simulink model "oxigeno"  (Simulink 7.5)
settings: Solver=ode45  StartTime=0.0  StopTime=10.0  RelTol=1e-3
settings Model: Creator=My Laptop  LastModifiedBy=My Laptop

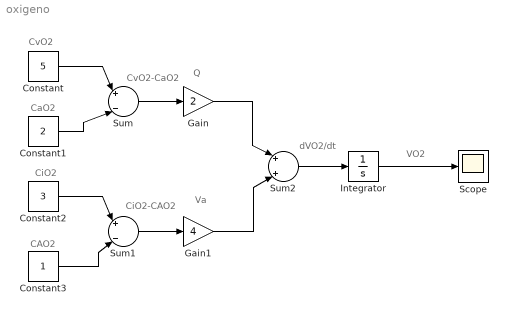
== system oxigeno ==
  note: dVO2/dt
  note: VO2
  note: CvO2
  note: CaO2
  note: CiO2
  note: CAO2
  note: Q
  note: Va
  note: CvO2-CaO2
  note: CiO2-CAO2
  Constant : Constant  Value=5  OutDataType=fixdt(1, 16)  OutScaling=2^0
  Constant1 : Constant  Value=2  OutDataType=fixdt(1, 16)  OutScaling=2^0
  Constant2 : Constant  Value=3  OutDataType=fixdt(1, 16)  OutScaling=2^0
  Constant3 : Constant  OutDataType=fixdt(1, 16)  OutScaling=2^0
  Gain : Gain  Gain=2  ParameterDataType=fixdt(1, 16)  ParameterScaling=2^0  OutDataType=fixdt(1, 16)  OutScaling=2^0
  Gain1 : Gain  Gain=4  ParameterDataType=fixdt(1, 16)  ParameterScaling=2^0  OutDataType=fixdt(1, 16)  OutScaling=2^0
  Integrator : Integrator  InitialCondition=50
  Scope : Scope
  Sum : Sum  Inputs=|+|-|  OutDataType=fixdt(1, 16)  OutScaling=2^0
  Sum1 : Sum  Inputs=|+|-|  OutDataType=fixdt(1, 16)  OutScaling=2^0
  Sum2 : Sum  Inputs=|+|+|  OutDataType=fixdt(1, 16)  OutScaling=2^0
  wires:
  Integrator/1 -> Scope/1
  Sum2/1 -> Integrator/1
  Gain/1 -> Sum2/1
  Gain1/1 -> Sum2/2
  Sum/1 -> Gain/1
  Sum1/1 -> Gain1/1
  Constant/1 -> Sum/1
  Constant1/1 -> Sum/2
  Constant3/1 -> Sum1/2
  Constant2/1 -> Sum1/1
